simulink model "kadai3"  (R2022a)
settings: Solver=VariableStepAuto  StartTime=0.0  StopTime=30.0  RelTol=1e-3
settings Model: Creator=mluser  LastModifiedBy=mluser

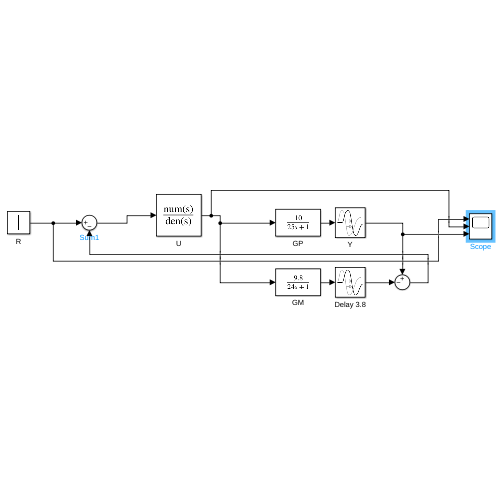
[thumbnail: Simulink's stored preview of the top-level diagram]
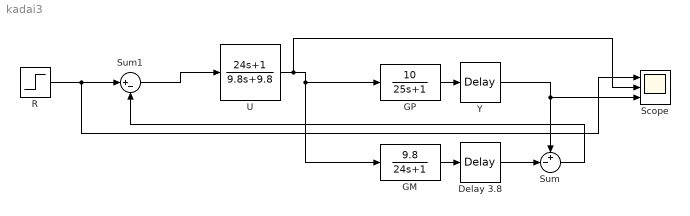
== system kadai3 ==
  Delay 3.8 : TransportDelay  DelayTime=3.8
  GM : TransferFcn  Numerator=[9.8]  Denominator=[24 1]
  GP : TransferFcn  Numerator=[10]  Denominator=[25 1]
  R : Step  Time=10  SampleTime=0
  Scope : Scope  NumInputPorts=3
  Sum : Sum  Inputs=+-|
  Sum1 : Sum  Inputs=|+-
  U : TransferFcn  Numerator=[24 1]  Denominator=[9.8 9.8]
  Y : TransportDelay  DelayTime=4
  wires:
  Sum1/1 -> U/1
  Y/1 -> Scope/3, Sum/1
  GP/1 -> Y/1
  GM/1 -> Delay 3.8/1
  Delay 3.8/1 -> Sum/2
  U/1 -> Scope/2, GM/1, GP/1
  Sum/1 -> Sum1/2
  R/1 -> Scope/1, Sum1/1
